simulink model "LsComp_TrqCalc"  (R2016b)
settings: configuration reference "CodeGenConfigSet" (kept outside this file)
values from neighbouring files (symbols this model uses):
  CoVeh_trqDesCompNoFl_C = Calibration.Parameter    [init_LsComp_TrqCalc.m]
  CoVeh_trqDesCompVeh_C = Calibration.Parameter    [init_LsComp_TrqCalc.m]
settings Model: Creator=Wollf  LastModifiedBy=Wollf
settings ConfigSetRef: SourceLocation=Base Workspace

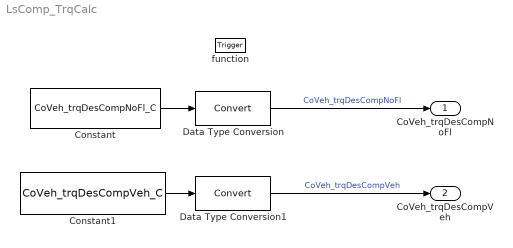
== system LsComp_TrqCalc ==
  function : TriggerPort  TriggerType=function-call  VariantControl=Variant
  Constant : Constant  Value=CoVeh_trqDesCompNoFl_C
  Constant1 : Constant  Value=CoVeh_trqDesCompVeh_C
  Data Type Conversion : DataTypeConversion
  Data Type Conversion1 : DataTypeConversion
  CoVeh_trqDesCompNoFl : Outport  Tag=Nm  Description=compensation torque with the shares,which not slur by the drive behaviour filter  OutMin=-3000  OutMax=3000  OutDataTypeStr=Trq_Nm
  CoVeh_trqDesCompVeh : Outport  Tag=Nm  Description=Signal for compensation correction of wheel torque level (signal 1)  Port=2  OutMin=-3000  OutMax=3000  OutDataTypeStr=Trq_Nm
  wires:
  Constant/1 -> Data Type Conversion/1
  Data Type Conversion/1 -> CoVeh_trqDesCompNoFl/1  "CoVeh_trqDesCompNoFl"
  Constant1/1 -> Data Type Conversion1/1
  Data Type Conversion1/1 -> CoVeh_trqDesCompVeh/1  "CoVeh_trqDesCompVeh"
